simulink model "RealLifeTrainModel"  (R2024a)
settings: Solver=ode1  StartTime=0.0  StopTime=Inf  FixedStep=0.001  RelTol=1e-3
PostLoadFcn:
  | , if any(exist('dsrtsu_mdlpostloadfcn', 'file') ~= 0), dsrtsu_mdlpostloadfcn('Execute', bdroot); end,
InitFcn:
  | , if any(exist('rtifpga_mdlclblib', 'file') ~= 0), rtifpga_mdlclblib('Init', bdroot); end,
undefined symbols (not defined in the file): DiscIntNeverNeededParam
libraries: deeplib x29, svdutilitieslib x28, simulink x8, eeGeneralControl x8, rti1202lib_adc_class1 x6, rti1202serlib x5, spsEdgeDetectorLib x5, rtiemclib x2, rti1202lib_dac_class1 x1
(part 5 of 8)

== system RealLifeTrainModel/ContractionMetricFilterSystem3/Calc_A_B/Calc_A_Grad/IndidualGrad6 ==
  State : Inport
  Position : Inport  Port=2
  StartValue : Inport  Port=3
  Data Type Conversion2 : DataTypeConversion  OutDataTypeStr=single  SaturateOnIntegerOverflow=off  RndMeth=Floor
  Data Type Conversion4 : DataTypeConversion  OutDataTypeStr=single  SaturateOnIntegerOverflow=off  RndMeth=Floor
  DynamicsConvert : MATLAB Function  TreatAsAtomicUnit=on
  MATLAB Function2 : MATLAB Function  TreatAsAtomicUnit=on
  MATLAB Function5 : MATLAB Function  TreatAsAtomicUnit=on
  Reshape : Reshape  OutputDimensionality=Customize  OutputDimensions=[8,1]
  Reshape1 : Reshape  OutputDimensionality=Customize  OutputDimensions=[8,1]
  Reshape2 : Reshape  OutputDimensionality=Customize  OutputDimensions=[8,1]
  SubsystemModel : Subsystem
  Sum4 : Sum  Inputs=|++
  Grad : Outport
  wires:
  [GradConst] -> MATLAB Function5/3(const)
  Sum4/1 -> Data Type Conversion2/1
  [GradConst] -> MATLAB Function2/1(u)
  State/1 -> Sum4/1
  MATLAB Function2/1(y) -> Sum4/2
  Position/1 -> MATLAB Function2/2(pos)
  MATLAB Function5/1(y) -> Reshape2/1
  StartValue/1 -> Reshape1/1
  Data Type Conversion2/1 -> SubsystemModel/1(u), DynamicsConvert/1(x)
  SubsystemModel/1(y) -> Data Type Conversion4/1
  [DiscreteContinousMode] -> DynamicsConvert/3(useDerivative)
  DynamicsConvert/1(dstate) -> Reshape/1
  Data Type Conversion4/1 -> DynamicsConvert/2(y_model)
  Reshape/1 -> MATLAB Function5/1(u1)
  Reshape1/1 -> MATLAB Function5/2(u2)
  Reshape2/1 -> Grad/1

== system RealLifeTrainModel/ContractionMetricFilterSystem3/Calc_A_B/Calc_A_Grad/IndidualGrad7 ==
  State : Inport
  Position : Inport  Port=2
  StartValue : Inport  Port=3
  Data Type Conversion2 : DataTypeConversion  OutDataTypeStr=single  SaturateOnIntegerOverflow=off  RndMeth=Floor
  Data Type Conversion4 : DataTypeConversion  OutDataTypeStr=single  SaturateOnIntegerOverflow=off  RndMeth=Floor
  DynamicsConvert : MATLAB Function  TreatAsAtomicUnit=on
  MATLAB Function2 : MATLAB Function  TreatAsAtomicUnit=on
  MATLAB Function5 : MATLAB Function  TreatAsAtomicUnit=on
  Reshape : Reshape  OutputDimensionality=Customize  OutputDimensions=[8,1]
  Reshape1 : Reshape  OutputDimensionality=Customize  OutputDimensions=[8,1]
  Reshape2 : Reshape  OutputDimensionality=Customize  OutputDimensions=[8,1]
  SubsystemModel : Subsystem
  Sum4 : Sum  Inputs=|++
  Grad : Outport
  wires:
  [GradConst] -> MATLAB Function5/3(const)
  Sum4/1 -> Data Type Conversion2/1
  [GradConst] -> MATLAB Function2/1(u)
  State/1 -> Sum4/1
  MATLAB Function2/1(y) -> Sum4/2
  Position/1 -> MATLAB Function2/2(pos)
  MATLAB Function5/1(y) -> Reshape2/1
  StartValue/1 -> Reshape1/1
  Data Type Conversion2/1 -> SubsystemModel/1(u), DynamicsConvert/1(x)
  SubsystemModel/1(y) -> Data Type Conversion4/1
  [DiscreteContinousMode] -> DynamicsConvert/3(useDerivative)
  Data Type Conversion4/1 -> DynamicsConvert/2(y_model)
  DynamicsConvert/1(dstate) -> Reshape/1
  Reshape/1 -> MATLAB Function5/1(u1)
  Reshape1/1 -> MATLAB Function5/2(u2)
  Reshape2/1 -> Grad/1

== system RealLifeTrainModel/ContractionMetricFilterSystem3/Calc_A_B/Calc_A_Grad/IndidualGrad8 ==
  State : Inport
  Position : Inport  Port=2
  StartValue : Inport  Port=3
  Data Type Conversion2 : DataTypeConversion  OutDataTypeStr=single  SaturateOnIntegerOverflow=off  RndMeth=Floor
  Data Type Conversion4 : DataTypeConversion  OutDataTypeStr=single  SaturateOnIntegerOverflow=off  RndMeth=Floor
  DynamicsConvert1 : MATLAB Function  TreatAsAtomicUnit=on
  MATLAB Function2 : MATLAB Function  TreatAsAtomicUnit=on
  MATLAB Function5 : MATLAB Function  TreatAsAtomicUnit=on
  Reshape : Reshape  OutputDimensionality=Customize  OutputDimensions=[8,1]
  Reshape1 : Reshape  OutputDimensionality=Customize  OutputDimensions=[8,1]
  Reshape2 : Reshape  OutputDimensionality=Customize  OutputDimensions=[8,1]
  SubsystemModel : Subsystem
  Sum4 : Sum  Inputs=|++
  Grad : Outport
  wires:
  [GradConst] -> MATLAB Function5/3(const)
  Sum4/1 -> Data Type Conversion2/1
  [GradConst] -> MATLAB Function2/1(u)
  State/1 -> Sum4/1
  MATLAB Function2/1(y) -> Sum4/2
  Position/1 -> MATLAB Function2/2(pos)
  StartValue/1 -> Reshape2/1
  Data Type Conversion2/1 -> SubsystemModel/1(u), DynamicsConvert1/1(x)
  SubsystemModel/1(y) -> Data Type Conversion4/1
  [DiscreteContinousMode] -> DynamicsConvert1/3(useDerivative)
  Data Type Conversion4/1 -> DynamicsConvert1/2(y_model)
  DynamicsConvert1/1(dstate) -> Reshape1/1
  MATLAB Function5/1(y) -> Reshape/1
  Reshape/1 -> Grad/1
  Reshape1/1 -> MATLAB Function5/1(u1)
  Reshape2/1 -> MATLAB Function5/2(u2)

== system RealLifeTrainModel/ContractionMetricFilterSystem3/Calc_A_B/Calc_A_Grad/SubsystemModel ==
  u : Inport
  Denormalize : MATLAB Function  TreatAsAtomicUnit=on
  Normalize : MATLAB Function  TreatAsAtomicUnit=on
  PredictModel : deeplib/Predict  Network=Network from MAT-file  NetworkFunction=squeezenet  NetworkFilePath=C:\Users\ic2d\Documents\GitHub\dSpace_Controllers_legged\model_1.mat  MiniBatchSize=128  InputDataFormats={'input', 'BC';}  Predictions=on  Activations={}  ForceInterpretedSim=off  EnableDLNetwork=on  LastKnownNetworkFilePath='C:\Users\ic2d\Documents\GitHub\dSpace_Controllers_legged\model_1.mat'  LastKnownNetworkTimeStamp=739864.429490740760229527950286865234375
  PredictModel1 : deeplib/Predict  Network=Network from MAT-file  NetworkFunction=squeezenet  NetworkFilePath=C:\Users\ic2d\Documents\GitHub\dSpace_Controllers_legged\model_2.mat  MiniBatchSize=128  InputDataFormats={'input', 'BC';}  Predictions=on  Activations={}  ForceInterpretedSim=off  EnableDLNetwork=on  LastKnownNetworkFilePath='C:\Users\ic2d\Documents\GitHub\dSpace_Controllers_legged\model_2.mat'  LastKnownNetworkTimeStamp=739864.429490740760229527950286865234375
  Product : Product
  Scope : Scope
  Square : Math  Operator=square
  Subsystem : Subsystem
  Subsystem1 : Subsystem
  Sum : Sum  Inputs=|++
  Transpose : Math  Operator=transpose
  y : Outport
  wires:
  PredictModel1/1 -> Square/1
  Square/1 -> Product/1
  Denormalize/1(y) -> y/1
  PredictModel/1 -> Sum/1
  Product/1 -> Sum/2
  Sum/1 -> Denormalize/1(u)
  u/1 -> Normalize/1(u)
  Normalize/1(y) -> Subsystem1/1(In1), Scope/1, Subsystem/1(In1)
  Subsystem1/1(Out1) -> Product/2
  Transpose/1 -> PredictModel1/1, PredictModel/1
  Subsystem/1(Out1) -> Transpose/1

== system RealLifeTrainModel/RTI Data/RTI Data Store/RTI Data Store/RTI Data Store ==
  RTI Data Store : Subsystem  mask(RTI_DATA_STORE){}
      mask help:
      | RTI Data Store Block. This block is used by RTI to store internal model dependent data. Deleting this block will result in data loss.
      |
      | NEVER DELETE, COPY, OR MODIFY THIS BLOCK!
      mask Help:
      | RTI Data Store Block. This block is used by RTI to store internal model dependent data. Deleting this block will result in data loss.
      | 
      | NEVER DELETE, COPY, OR MODIFY THIS BLOCK!
      mask Display: text(0.5, 0.5, ' ', 'HorizontalAlignment', 'center');

== system RealLifeTrainModel/ContractionMetricFilterSystem3/Calc_A_B/Calc_A_Grad/IndidualGrad1/SubsystemModel ==
  u : Inport
  Denormalize : MATLAB Function  TreatAsAtomicUnit=on
  Normalize : MATLAB Function  TreatAsAtomicUnit=on
  PredictModel : deeplib/Predict  Network=Network from MAT-file  NetworkFunction=squeezenet  NetworkFilePath=C:\Users\ic2d\Documents\GitHub\dSpace_Controllers_legged\model_1.mat  MiniBatchSize=128  InputDataFormats={'input', 'BC';}  Predictions=on  Activations={}  ForceInterpretedSim=off  EnableDLNetwork=on  LastKnownNetworkFilePath='C:\Users\ic2d\Documents\GitHub\dSpace_Controllers_legged\model_1.mat'  LastKnownNetworkTimeStamp=739864.429490740760229527950286865234375
  PredictModel1 : deeplib/Predict  Network=Network from MAT-file  NetworkFunction=squeezenet  NetworkFilePath=C:\Users\ic2d\Documents\GitHub\dSpace_Controllers_legged\model_2.mat  MiniBatchSize=128  InputDataFormats={'input', 'BC';}  Predictions=on  Activations={}  ForceInterpretedSim=off  EnableDLNetwork=on  LastKnownNetworkFilePath='C:\Users\ic2d\Documents\GitHub\dSpace_Controllers_legged\model_2.mat'  LastKnownNetworkTimeStamp=739864.429490740760229527950286865234375
  Product : Product
  Square : Math  Operator=square
  Subsystem : Subsystem
  Subsystem1 : Subsystem
  Sum : Sum  Inputs=|++
  Transpose : Math  Operator=transpose
  y : Outport
  wires:
  PredictModel1/1 -> Square/1
  Square/1 -> Product/1
  Denormalize/1(y) -> y/1
  PredictModel/1 -> Sum/1
  Product/1 -> Sum/2
  Sum/1 -> Denormalize/1(u)
  u/1 -> Normalize/1(u)
  Normalize/1(y) -> Subsystem1/1(In1), Subsystem/1(In1)
  Subsystem/1(Out1) -> Transpose/1
  Subsystem1/1(Out1) -> Product/2
  Transpose/1 -> PredictModel1/1, PredictModel/1

== system RealLifeTrainModel/ContractionMetricFilterSystem3/Calc_A_B/Calc_A_Grad/IndidualGrad10/SubsystemModel ==
  u : Inport
  Denormalize : MATLAB Function  TreatAsAtomicUnit=on
  Normalize : MATLAB Function  TreatAsAtomicUnit=on
  PredictModel : deeplib/Predict  Network=Network from MAT-file  NetworkFunction=squeezenet  NetworkFilePath=C:\Users\ic2d\Documents\GitHub\dSpace_Controllers_legged\model_1.mat  MiniBatchSize=128  InputDataFormats={'input', 'BC';}  Predictions=on  Activations={}  ForceInterpretedSim=off  EnableDLNetwork=on  LastKnownNetworkFilePath='C:\Users\ic2d\Documents\GitHub\dSpace_Controllers_legged\model_1.mat'  LastKnownNetworkTimeStamp=739864.429490740760229527950286865234375
  PredictModel1 : deeplib/Predict  Network=Network from MAT-file  NetworkFunction=squeezenet  NetworkFilePath=C:\Users\ic2d\Documents\GitHub\dSpace_Controllers_legged\model_2.mat  MiniBatchSize=128  InputDataFormats={'input', 'BC';}  Predictions=on  Activations={}  ForceInterpretedSim=off  EnableDLNetwork=on  LastKnownNetworkFilePath='C:\Users\ic2d\Documents\GitHub\dSpace_Controllers_legged\model_2.mat'  LastKnownNetworkTimeStamp=739864.429490740760229527950286865234375
  Product : Product
  Square : Math  Operator=square
  Subsystem : Subsystem
  Subsystem1 : Subsystem
  Sum : Sum  Inputs=|++
  Transpose : Math  Operator=transpose
  y : Outport
  wires:
  PredictModel1/1 -> Square/1
  Square/1 -> Product/1
  Denormalize/1(y) -> y/1
  PredictModel/1 -> Sum/1
  Product/1 -> Sum/2
  Sum/1 -> Denormalize/1(u)
  u/1 -> Normalize/1(u)
  Normalize/1(y) -> Subsystem1/1(In1), Subsystem/1(In1)
  Subsystem/1(Out1) -> Transpose/1
  Subsystem1/1(Out1) -> Product/2
  Transpose/1 -> PredictModel1/1, PredictModel/1

== system RealLifeTrainModel/ContractionMetricFilterSystem3/Calc_A_B/Calc_A_Grad/IndidualGrad2/SubsystemModel ==
  u : Inport
  Denormalize : MATLAB Function  TreatAsAtomicUnit=on
  Normalize : MATLAB Function  TreatAsAtomicUnit=on
  PredictModel : deeplib/Predict  Network=Network from MAT-file  NetworkFunction=squeezenet  NetworkFilePath=C:\Users\ic2d\Documents\GitHub\dSpace_Controllers_legged\model_1.mat  MiniBatchSize=128  InputDataFormats={'input', 'BC';}  Predictions=on  Activations={}  ForceInterpretedSim=off  EnableDLNetwork=on  LastKnownNetworkFilePath='C:\Users\ic2d\Documents\GitHub\dSpace_Controllers_legged\model_1.mat'  LastKnownNetworkTimeStamp=739864.429490740760229527950286865234375
  PredictModel1 : deeplib/Predict  Network=Network from MAT-file  NetworkFunction=squeezenet  NetworkFilePath=C:\Users\ic2d\Documents\GitHub\dSpace_Controllers_legged\model_2.mat  MiniBatchSize=128  InputDataFormats={'input', 'BC';}  Predictions=on  Activations={}  ForceInterpretedSim=off  EnableDLNetwork=on  LastKnownNetworkFilePath='C:\Users\ic2d\Documents\GitHub\dSpace_Controllers_legged\model_2.mat'  LastKnownNetworkTimeStamp=739864.429490740760229527950286865234375
  Product : Product
  Square : Math  Operator=square
  Subsystem : Subsystem
  Subsystem1 : Subsystem
  Sum : Sum  Inputs=|++
  Transpose : Math  Operator=transpose
  y : Outport
  wires:
  PredictModel1/1 -> Square/1
  Square/1 -> Product/1
  Denormalize/1(y) -> y/1
  PredictModel/1 -> Sum/1
  Product/1 -> Sum/2
  Sum/1 -> Denormalize/1(u)
  u/1 -> Normalize/1(u)
  Normalize/1(y) -> Subsystem1/1(In1), Subsystem/1(In1)
  Subsystem/1(Out1) -> Transpose/1
  Subsystem1/1(Out1) -> Product/2
  Transpose/1 -> PredictModel1/1, PredictModel/1

== system RealLifeTrainModel/ContractionMetricFilterSystem3/Calc_A_B/Calc_A_Grad/IndidualGrad3/SubsystemModel ==
  u : Inport
  Denormalize : MATLAB Function  TreatAsAtomicUnit=on
  Normalize : MATLAB Function  TreatAsAtomicUnit=on
  PredictModel : deeplib/Predict  Network=Network from MAT-file  NetworkFunction=squeezenet  NetworkFilePath=C:\Users\ic2d\Documents\GitHub\dSpace_Controllers_legged\model_1.mat  MiniBatchSize=128  InputDataFormats={'input', 'BC';}  Predictions=on  Activations={}  ForceInterpretedSim=off  EnableDLNetwork=on  LastKnownNetworkFilePath='C:\Users\ic2d\Documents\GitHub\dSpace_Controllers_legged\model_1.mat'  LastKnownNetworkTimeStamp=739864.429490740760229527950286865234375
  PredictModel1 : deeplib/Predict  Network=Network from MAT-file  NetworkFunction=squeezenet  NetworkFilePath=C:\Users\ic2d\Documents\GitHub\dSpace_Controllers_legged\model_2.mat  MiniBatchSize=128  InputDataFormats={'input', 'BC';}  Predictions=on  Activations={}  ForceInterpretedSim=off  EnableDLNetwork=on  LastKnownNetworkFilePath='C:\Users\ic2d\Documents\GitHub\dSpace_Controllers_legged\model_2.mat'  LastKnownNetworkTimeStamp=739864.429490740760229527950286865234375
  Product : Product
  Square : Math  Operator=square
  Subsystem : Subsystem
  Subsystem1 : Subsystem
  Sum : Sum  Inputs=|++
  Transpose : Math  Operator=transpose
  y : Outport
  wires:
  PredictModel1/1 -> Square/1
  Square/1 -> Product/1
  Denormalize/1(y) -> y/1
  PredictModel/1 -> Sum/1
  Product/1 -> Sum/2
  Sum/1 -> Denormalize/1(u)
  u/1 -> Normalize/1(u)
  Normalize/1(y) -> Subsystem1/1(In1), Subsystem/1(In1)
  Subsystem/1(Out1) -> Transpose/1
  Subsystem1/1(Out1) -> Product/2
  Transpose/1 -> PredictModel1/1, PredictModel/1

== system RealLifeTrainModel/ContractionMetricFilterSystem3/Calc_A_B/Calc_A_Grad/IndidualGrad4/SubsystemModel ==
  u : Inport
  Denormalize : MATLAB Function  TreatAsAtomicUnit=on
  Normalize : MATLAB Function  TreatAsAtomicUnit=on
  PredictModel : deeplib/Predict  Network=Network from MAT-file  NetworkFunction=squeezenet  NetworkFilePath=C:\Users\ic2d\Documents\GitHub\dSpace_Controllers_legged\model_1.mat  MiniBatchSize=128  InputDataFormats={'input', 'BC';}  Predictions=on  Activations={}  ForceInterpretedSim=off  EnableDLNetwork=on  LastKnownNetworkFilePath='C:\Users\ic2d\Documents\GitHub\dSpace_Controllers_legged\model_1.mat'  LastKnownNetworkTimeStamp=739864.429490740760229527950286865234375
  PredictModel1 : deeplib/Predict  Network=Network from MAT-file  NetworkFunction=squeezenet  NetworkFilePath=C:\Users\ic2d\Documents\GitHub\dSpace_Controllers_legged\model_2.mat  MiniBatchSize=128  InputDataFormats={'input', 'BC';}  Predictions=on  Activations={}  ForceInterpretedSim=off  EnableDLNetwork=on  LastKnownNetworkFilePath='C:\Users\ic2d\Documents\GitHub\dSpace_Controllers_legged\model_2.mat'  LastKnownNetworkTimeStamp=739864.429490740760229527950286865234375
  Product : Product
  Square : Math  Operator=square
  Subsystem : Subsystem
  Subsystem1 : Subsystem
  Sum : Sum  Inputs=|++
  Transpose : Math  Operator=transpose
  y : Outport
  wires:
  PredictModel1/1 -> Square/1
  Square/1 -> Product/1
  Denormalize/1(y) -> y/1
  PredictModel/1 -> Sum/1
  Product/1 -> Sum/2
  Sum/1 -> Denormalize/1(u)
  u/1 -> Normalize/1(u)
  Normalize/1(y) -> Subsystem1/1(In1), Subsystem/1(In1)
  Subsystem/1(Out1) -> Transpose/1
  Subsystem1/1(Out1) -> Product/2
  Transpose/1 -> PredictModel1/1, PredictModel/1

== system RealLifeTrainModel/ContractionMetricFilterSystem3/Calc_A_B/Calc_A_Grad/IndidualGrad5/SubsystemModel ==
  u : Inport
  Denormalize : MATLAB Function  TreatAsAtomicUnit=on
  Normalize : MATLAB Function  TreatAsAtomicUnit=on
  PredictModel : deeplib/Predict  Network=Network from MAT-file  NetworkFunction=squeezenet  NetworkFilePath=C:\Users\ic2d\Documents\GitHub\dSpace_Controllers_legged\model_1.mat  MiniBatchSize=128  InputDataFormats={'input', 'BC';}  Predictions=on  Activations={}  ForceInterpretedSim=off  EnableDLNetwork=on  LastKnownNetworkFilePath='C:\Users\ic2d\Documents\GitHub\dSpace_Controllers_legged\model_1.mat'  LastKnownNetworkTimeStamp=739864.429490740760229527950286865234375
  PredictModel1 : deeplib/Predict  Network=Network from MAT-file  NetworkFunction=squeezenet  NetworkFilePath=C:\Users\ic2d\Documents\GitHub\dSpace_Controllers_legged\model_2.mat  MiniBatchSize=128  InputDataFormats={'input', 'BC';}  Predictions=on  Activations={}  ForceInterpretedSim=off  EnableDLNetwork=on  LastKnownNetworkFilePath='C:\Users\ic2d\Documents\GitHub\dSpace_Controllers_legged\model_2.mat'  LastKnownNetworkTimeStamp=739864.429490740760229527950286865234375
  Product : Product
  Square : Math  Operator=square
  Subsystem : Subsystem
  Subsystem1 : Subsystem
  Sum : Sum  Inputs=|++
  Transpose : Math  Operator=transpose
  y : Outport
  wires:
  PredictModel1/1 -> Square/1
  Square/1 -> Product/1
  Denormalize/1(y) -> y/1
  PredictModel/1 -> Sum/1
  Product/1 -> Sum/2
  Sum/1 -> Denormalize/1(u)
  u/1 -> Normalize/1(u)
  Normalize/1(y) -> Subsystem1/1(In1), Subsystem/1(In1)
  Subsystem/1(Out1) -> Transpose/1
  Subsystem1/1(Out1) -> Product/2
  Transpose/1 -> PredictModel1/1, PredictModel/1

== system RealLifeTrainModel/ContractionMetricFilterSystem3/Calc_A_B/Calc_A_Grad/IndidualGrad6/SubsystemModel ==
  u : Inport
  Denormalize : MATLAB Function  TreatAsAtomicUnit=on
  Normalize : MATLAB Function  TreatAsAtomicUnit=on
  PredictModel : deeplib/Predict  Network=Network from MAT-file  NetworkFunction=squeezenet  NetworkFilePath=C:\Users\ic2d\Documents\GitHub\dSpace_Controllers_legged\model_1.mat  MiniBatchSize=128  InputDataFormats={'input', 'BC';}  Predictions=on  Activations={}  ForceInterpretedSim=off  EnableDLNetwork=on  LastKnownNetworkFilePath='C:\Users\ic2d\Documents\GitHub\dSpace_Controllers_legged\model_1.mat'  LastKnownNetworkTimeStamp=739864.429490740760229527950286865234375
  PredictModel1 : deeplib/Predict  Network=Network from MAT-file  NetworkFunction=squeezenet  NetworkFilePath=C:\Users\ic2d\Documents\GitHub\dSpace_Controllers_legged\model_2.mat  MiniBatchSize=128  InputDataFormats={'input', 'BC';}  Predictions=on  Activations={}  ForceInterpretedSim=off  EnableDLNetwork=on  LastKnownNetworkFilePath='C:\Users\ic2d\Documents\GitHub\dSpace_Controllers_legged\model_2.mat'  LastKnownNetworkTimeStamp=739864.429490740760229527950286865234375
  Product : Product
  Square : Math  Operator=square
  Subsystem : Subsystem
  Subsystem1 : Subsystem
  Sum : Sum  Inputs=|++
  Transpose : Math  Operator=transpose
  y : Outport
  wires:
  PredictModel1/1 -> Square/1
  Square/1 -> Product/1
  Denormalize/1(y) -> y/1
  PredictModel/1 -> Sum/1
  Product/1 -> Sum/2
  Sum/1 -> Denormalize/1(u)
  u/1 -> Normalize/1(u)
  Normalize/1(y) -> Subsystem1/1(In1), Subsystem/1(In1)
  Subsystem/1(Out1) -> Transpose/1
  Subsystem1/1(Out1) -> Product/2
  Transpose/1 -> PredictModel1/1, PredictModel/1

== system RealLifeTrainModel/ContractionMetricFilterSystem3/Calc_A_B/Calc_A_Grad/IndidualGrad7/SubsystemModel ==
  u : Inport
  Denormalize : MATLAB Function  TreatAsAtomicUnit=on
  Normalize : MATLAB Function  TreatAsAtomicUnit=on
  PredictModel : deeplib/Predict  Network=Network from MAT-file  NetworkFunction=squeezenet  NetworkFilePath=C:\Users\ic2d\Documents\GitHub\dSpace_Controllers_legged\model_1.mat  MiniBatchSize=128  InputDataFormats={'input', 'BC';}  Predictions=on  Activations={}  ForceInterpretedSim=off  EnableDLNetwork=on  LastKnownNetworkFilePath='C:\Users\ic2d\Documents\GitHub\dSpace_Controllers_legged\model_1.mat'  LastKnownNetworkTimeStamp=739864.429490740760229527950286865234375
  PredictModel1 : deeplib/Predict  Network=Network from MAT-file  NetworkFunction=squeezenet  NetworkFilePath=C:\Users\ic2d\Documents\GitHub\dSpace_Controllers_legged\model_2.mat  MiniBatchSize=128  InputDataFormats={'input', 'BC';}  Predictions=on  Activations={}  ForceInterpretedSim=off  EnableDLNetwork=on  LastKnownNetworkFilePath='C:\Users\ic2d\Documents\GitHub\dSpace_Controllers_legged\model_2.mat'  LastKnownNetworkTimeStamp=739864.429490740760229527950286865234375
  Product : Product
  Square : Math  Operator=square
  Subsystem : Subsystem
  Subsystem1 : Subsystem
  Sum : Sum  Inputs=|++
  Transpose : Math  Operator=transpose
  y : Outport
  wires:
  PredictModel1/1 -> Square/1
  Square/1 -> Product/1
  Denormalize/1(y) -> y/1
  PredictModel/1 -> Sum/1
  Product/1 -> Sum/2
  Sum/1 -> Denormalize/1(u)
  u/1 -> Normalize/1(u)
  Normalize/1(y) -> Subsystem1/1(In1), Subsystem/1(In1)
  Subsystem/1(Out1) -> Transpose/1
  Subsystem1/1(Out1) -> Product/2
  Transpose/1 -> PredictModel1/1, PredictModel/1

== system RealLifeTrainModel/ContractionMetricFilterSystem3/Calc_A_B/Calc_A_Grad/IndidualGrad8/SubsystemModel ==
  u : Inport
  Denormalize : MATLAB Function  TreatAsAtomicUnit=on
  Normalize : MATLAB Function  TreatAsAtomicUnit=on
  PredictModel : deeplib/Predict  Network=Network from MAT-file  NetworkFunction=squeezenet  NetworkFilePath=C:\Users\ic2d\Documents\GitHub\dSpace_Controllers_legged\model_1.mat  MiniBatchSize=128  InputDataFormats={'input', 'BC';}  Predictions=on  Activations={}  ForceInterpretedSim=off  EnableDLNetwork=on  LastKnownNetworkFilePath='C:\Users\ic2d\Documents\GitHub\dSpace_Controllers_legged\model_1.mat'  LastKnownNetworkTimeStamp=739864.429490740760229527950286865234375
  PredictModel1 : deeplib/Predict  Network=Network from MAT-file  NetworkFunction=squeezenet  NetworkFilePath=C:\Users\ic2d\Documents\GitHub\dSpace_Controllers_legged\model_2.mat  MiniBatchSize=128  InputDataFormats={'input', 'BC';}  Predictions=on  Activations={}  ForceInterpretedSim=off  EnableDLNetwork=on  LastKnownNetworkFilePath='C:\Users\ic2d\Documents\GitHub\dSpace_Controllers_legged\model_2.mat'  LastKnownNetworkTimeStamp=739864.429490740760229527950286865234375
  Product : Product
  Square : Math  Operator=square
  Subsystem : Subsystem
  Subsystem1 : Subsystem
  Sum : Sum  Inputs=|++
  Transpose : Math  Operator=transpose
  y : Outport
  wires:
  PredictModel1/1 -> Square/1
  Square/1 -> Product/1
  Denormalize/1(y) -> y/1
  PredictModel/1 -> Sum/1
  Product/1 -> Sum/2
  Sum/1 -> Denormalize/1(u)
  u/1 -> Normalize/1(u)
  Normalize/1(y) -> Subsystem1/1(In1), Subsystem/1(In1)
  Subsystem1/1(Out1) -> Product/2
  Subsystem/1(Out1) -> Transpose/1
  Transpose/1 -> PredictModel1/1, PredictModel/1

== system RealLifeTrainModel/ContractionMetricFilterSystem3/Calc_A_B/Calc_A_Grad/SubsystemModel/Subsystem ==
  In1 : Inport
  Demux : Demux  Outputs=9
  Mux : Mux  Inputs=8
  Out1 : Outport
  wires:
  In1/1 -> Demux/1
  Demux/1 -> Mux/1
  Demux/2 -> Mux/2
  Demux/3 -> Mux/3
  Demux/4 -> Mux/4
  Demux/5 -> Mux/5
  Demux/6 -> Mux/6
  Demux/7 -> Mux/7
  Demux/8 -> Mux/8
  Mux/1 -> Out1/1

== system RealLifeTrainModel/ContractionMetricFilterSystem3/Calc_A_B/Calc_A_Grad/SubsystemModel/Subsystem1 ==
  In1 : Inport
  Demux : Demux  Outputs=9
  Out1 : Outport
  wires:
  In1/1 -> Demux/1
  Demux/9 -> Out1/1

== system RealLifeTrainModel/RTI Data/RTI Data Store/RTI Data Store/RTI Data Store/RTI Data Store ==

== system RealLifeTrainModel/ContractionMetricFilterSystem3/Calc_A_B/Calc_A_Grad/IndidualGrad1/SubsystemModel/Subsystem ==
  In1 : Inport
  Demux : Demux  Outputs=9
  Mux : Mux  Inputs=8
  Out1 : Outport
  wires:
  In1/1 -> Demux/1
  Demux/1 -> Mux/1
  Demux/2 -> Mux/2
  Demux/3 -> Mux/3
  Demux/4 -> Mux/4
  Demux/5 -> Mux/5
  Demux/6 -> Mux/6
  Demux/7 -> Mux/7
  Demux/8 -> Mux/8
  Mux/1 -> Out1/1

== system RealLifeTrainModel/ContractionMetricFilterSystem3/Calc_A_B/Calc_A_Grad/IndidualGrad1/SubsystemModel/Subsystem1 ==
  In1 : Inport
  Demux : Demux  Outputs=9
  Out1 : Outport
  wires:
  In1/1 -> Demux/1
  Demux/9 -> Out1/1

== system RealLifeTrainModel/ContractionMetricFilterSystem3/Calc_A_B/Calc_A_Grad/IndidualGrad10/SubsystemModel/Subsystem ==
  In1 : Inport
  Demux : Demux  Outputs=9
  Mux : Mux  Inputs=8
  Out1 : Outport
  wires:
  In1/1 -> Demux/1
  Demux/1 -> Mux/1
  Demux/2 -> Mux/2
  Demux/3 -> Mux/3
  Demux/4 -> Mux/4
  Demux/5 -> Mux/5
  Demux/6 -> Mux/6
  Demux/7 -> Mux/7
  Demux/8 -> Mux/8
  Mux/1 -> Out1/1

== system RealLifeTrainModel/ContractionMetricFilterSystem3/Calc_A_B/Calc_A_Grad/IndidualGrad10/SubsystemModel/Subsystem1 ==
  In1 : Inport
  Demux : Demux  Outputs=9
  Out1 : Outport
  wires:
  In1/1 -> Demux/1
  Demux/9 -> Out1/1

== system RealLifeTrainModel/ContractionMetricFilterSystem3/Calc_A_B/Calc_A_Grad/IndidualGrad2/SubsystemModel/Subsystem ==
  In1 : Inport
  Demux : Demux  Outputs=9
  Mux : Mux  Inputs=8
  Out1 : Outport
  wires:
  In1/1 -> Demux/1
  Demux/1 -> Mux/1
  Demux/2 -> Mux/2
  Demux/3 -> Mux/3
  Demux/4 -> Mux/4
  Demux/5 -> Mux/5
  Demux/6 -> Mux/6
  Demux/7 -> Mux/7
  Demux/8 -> Mux/8
  Mux/1 -> Out1/1

== system RealLifeTrainModel/ContractionMetricFilterSystem3/Calc_A_B/Calc_A_Grad/IndidualGrad2/SubsystemModel/Subsystem1 ==
  In1 : Inport
  Demux : Demux  Outputs=9
  Out1 : Outport
  wires:
  In1/1 -> Demux/1
  Demux/9 -> Out1/1

== system RealLifeTrainModel/ContractionMetricFilterSystem3/Calc_A_B/Calc_A_Grad/IndidualGrad3/SubsystemModel/Subsystem ==
  In1 : Inport
  Demux : Demux  Outputs=9
  Mux : Mux  Inputs=8
  Out1 : Outport
  wires:
  In1/1 -> Demux/1
  Demux/1 -> Mux/1
  Demux/2 -> Mux/2
  Demux/3 -> Mux/3
  Demux/4 -> Mux/4
  Demux/5 -> Mux/5
  Demux/6 -> Mux/6
  Demux/7 -> Mux/7
  Demux/8 -> Mux/8
  Mux/1 -> Out1/1

== system RealLifeTrainModel/ContractionMetricFilterSystem3/Calc_A_B/Calc_A_Grad/IndidualGrad3/SubsystemModel/Subsystem1 ==
  In1 : Inport
  Demux : Demux  Outputs=9
  Out1 : Outport
  wires:
  In1/1 -> Demux/1
  Demux/9 -> Out1/1

== system RealLifeTrainModel/ContractionMetricFilterSystem3/Calc_A_B/Calc_A_Grad/IndidualGrad4/SubsystemModel/Subsystem ==
  In1 : Inport
  Demux : Demux  Outputs=9
  Mux : Mux  Inputs=8
  Out1 : Outport
  wires:
  In1/1 -> Demux/1
  Demux/1 -> Mux/1
  Demux/2 -> Mux/2
  Demux/3 -> Mux/3
  Demux/4 -> Mux/4
  Demux/5 -> Mux/5
  Demux/6 -> Mux/6
  Demux/7 -> Mux/7
  Demux/8 -> Mux/8
  Mux/1 -> Out1/1

== system RealLifeTrainModel/ContractionMetricFilterSystem3/Calc_A_B/Calc_A_Grad/IndidualGrad4/SubsystemModel/Subsystem1 ==
  In1 : Inport
  Demux : Demux  Outputs=9
  Out1 : Outport
  wires:
  In1/1 -> Demux/1
  Demux/9 -> Out1/1

== system RealLifeTrainModel/ContractionMetricFilterSystem3/Calc_A_B/Calc_A_Grad/IndidualGrad5/SubsystemModel/Subsystem ==
  In1 : Inport
  Demux : Demux  Outputs=9
  Mux : Mux  Inputs=8
  Out1 : Outport
  wires:
  In1/1 -> Demux/1
  Demux/1 -> Mux/1
  Demux/2 -> Mux/2
  Demux/3 -> Mux/3
  Demux/4 -> Mux/4
  Demux/5 -> Mux/5
  Demux/6 -> Mux/6
  Demux/7 -> Mux/7
  Demux/8 -> Mux/8
  Mux/1 -> Out1/1

== system RealLifeTrainModel/ContractionMetricFilterSystem3/Calc_A_B/Calc_A_Grad/IndidualGrad5/SubsystemModel/Subsystem1 ==
  In1 : Inport
  Demux : Demux  Outputs=9
  Out1 : Outport
  wires:
  In1/1 -> Demux/1
  Demux/9 -> Out1/1

== system RealLifeTrainModel/ContractionMetricFilterSystem3/Calc_A_B/Calc_A_Grad/IndidualGrad6/SubsystemModel/Subsystem ==
  In1 : Inport
  Demux : Demux  Outputs=9
  Mux : Mux  Inputs=8
  Out1 : Outport
  wires:
  In1/1 -> Demux/1
  Demux/1 -> Mux/1
  Demux/2 -> Mux/2
  Demux/3 -> Mux/3
  Demux/4 -> Mux/4
  Demux/5 -> Mux/5
  Demux/6 -> Mux/6
  Demux/7 -> Mux/7
  Demux/8 -> Mux/8
  Mux/1 -> Out1/1

== system RealLifeTrainModel/ContractionMetricFilterSystem3/Calc_A_B/Calc_A_Grad/IndidualGrad6/SubsystemModel/Subsystem1 ==
  In1 : Inport
  Demux : Demux  Outputs=9
  Out1 : Outport
  wires:
  In1/1 -> Demux/1
  Demux/9 -> Out1/1

== system RealLifeTrainModel/ContractionMetricFilterSystem3/Calc_A_B/Calc_A_Grad/IndidualGrad7/SubsystemModel/Subsystem ==
  In1 : Inport
  Demux : Demux  Outputs=9
  Mux : Mux  Inputs=8
  Out1 : Outport
  wires:
  In1/1 -> Demux/1
  Demux/1 -> Mux/1
  Demux/2 -> Mux/2
  Demux/3 -> Mux/3
  Demux/4 -> Mux/4
  Demux/5 -> Mux/5
  Demux/6 -> Mux/6
  Demux/7 -> Mux/7
  Demux/8 -> Mux/8
  Mux/1 -> Out1/1

== system RealLifeTrainModel/ContractionMetricFilterSystem3/Calc_A_B/Calc_A_Grad/IndidualGrad7/SubsystemModel/Subsystem1 ==
  In1 : Inport
  Demux : Demux  Outputs=9
  Out1 : Outport
  wires:
  In1/1 -> Demux/1
  Demux/9 -> Out1/1

== system RealLifeTrainModel/ContractionMetricFilterSystem3/Calc_A_B/Calc_A_Grad/IndidualGrad8/SubsystemModel/Subsystem ==
  In1 : Inport
  Demux : Demux  Outputs=9
  Mux : Mux  Inputs=8
  Out1 : Outport
  wires:
  In1/1 -> Demux/1
  Demux/1 -> Mux/1
  Demux/2 -> Mux/2
  Demux/3 -> Mux/3
  Demux/4 -> Mux/4
  Demux/5 -> Mux/5
  Demux/6 -> Mux/6
  Demux/7 -> Mux/7
  Demux/8 -> Mux/8
  Mux/1 -> Out1/1

== system RealLifeTrainModel/ContractionMetricFilterSystem3/Calc_A_B/Calc_A_Grad/IndidualGrad8/SubsystemModel/Subsystem1 ==
  In1 : Inport
  Demux : Demux  Outputs=9
  Out1 : Outport
  wires:
  In1/1 -> Demux/1
  Demux/9 -> Out1/1

== matlab function RealLifeTrainModel/ContractionMetricFilterSystem3/CalcK/IndidualGrad1/Policy_SS1/Policy ==
  data: u input; y output
function y = fcn(u)

y = (u)/2 + 0.5;

== matlab function RealLifeTrainModel/ContractionMetricFilterSystem3/CalcK/IndidualGrad1/Policy_SS1/SmoothFnc1 ==
  data: u input; y output; smooth input
function y = fcn(u,smooth)
persistent last_value;

if(isempty(last_value))
    last_value = 0
end

y = smooth*last_value + (1 - smooth)*u
last_value = u

== matlab function RealLifeTrainModel/RefStepFunction ==
  data: Time input; y output; Amp input; StartTime input; EndTime input
function y = fcn(Time,Amp,StartTime,EndTime)

if((Time - StartTime) < 5)
    y = 0;
elseif ((EndTime + StartTime - Time) < 5)
    y = 0;
else
    y = Amp;
end

== matlab function RealLifeTrainModel/ContractionMetricFilterSystem3/CalcK/IndidualGrad10/MATLAB Function2 ==
  data: u input; y output; pos input
function y = fcn(u,pos)

a = [0,0,0,0,0,0,0,0,0]

a(pos) = u

y = a;

== matlab function RealLifeTrainModel/ContractionMetricFilterSystem3/CalcK/IndidualGrad10/MATLAB Function5 ==
  data: u1 input; y output; u2 input; const input
function y = fcn(u1,u2,const)

y = (u1 - u2)/(const);

== matlab function RealLifeTrainModel/ContractionMetricFilterSystem3/CalcK/IndidualGrad10/Policy_SS1/Denormalize_Policy ==
  data: u input; y output
function y = fcn(u)

max_Fload =  569.629505294963
min_Fload = -610.339671010468

max_Fhyd = 729.261146885585
min_Fhyd = -777.489547410502

max_DFload = 123011.265014651
min_DFload = -142353.177843906

max_DFhyd = 219994.429294316
min_DFhyd = -270882.694509076

max_Pa = 12037835.3221229
min_Pa = 1849925.22965178

max_Pb = 14831789.6053956
min_Pb = 2808786.27887814

max_x = 0.082368752
min_x = 0.01990812

max_Dx = 0.682789396628826
min_Dx = -0.578996654196926

out = [1,1,1,1,1,1,1,1,1]

out(1) = (u(1))*(max_Fhyd - min_Fhyd) + min_Fhyd;

out(2) = (u(2))*(max_DFhyd - min_DFhyd) + min_DFhyd;

out(3) = (u(3))*(max_Fload - min_Fload) + min_Fload;

out(4) = (u(4))*(max_DFload - min_DFload) + min_DFload;

out(5) = (u(5))*(max_Pa - min_Pa) + min_Pa;

out(6) = (u(6))*(max_Pb - min_Pb) + min_Pb;

out(7) = (u(7))*(max_x - min_x) + min_x;

out(8) = (u(8))*(max_Dx - min_Dx) + min_Dx;

out(9) = (u(9))*(max_Fload - min_Fload) + min_Fload;


y = out;

== matlab function RealLifeTrainModel/ContractionMetricFilterSystem3/CalcK/IndidualGrad10/Policy_SS1/FLcontroller1 ==
  data: pid input; y output; f input; g input; dFref input; d input; flag_start input
function y = fcn(pid,f,g,dFref,d,flag_start)

if flag_start == 1
    y = (dFref + pid - f)/g - d;
else 
    y = 1;
end

== matlab function RealLifeTrainModel/ContractionMetricFilterSystem3/CalcK/IndidualGrad10/Policy_SS1/FunctionCalculateHydModel1 ==
  data: ixv input; f output; Pn input; Qn input; Un input; Vpl input; Ps input; Pt input; L_cyl input; Aa input; alfa input; c1 input; c2 input; Be input; flag_start input; data input; g output; force output
function [f,g,force] = fcn(ixv,Pn,Qn,Un,Vpl,Ps,Pt,L_cyl,Aa,alfa,c1,c2,Be,flag_start,data)
force = 0
if flag_start == 1
    Pa = data(5)
    Pb = data(6)
    xp = data(7)
    xpd = data(8)
    force = data(3)

    Kv = Qn/(Un*sqrt(Pn/2));
    
    Va = Vpl + Aa*xp;
    Vb = Vpl + (L_cyl - xp)*alfa*Aa;

    if(ixv >= 0)
        g = Be*Aa*Kv*( sign(Ps-Pa)*sqrt(abs(Ps-Pa))/Va + alfa*sign(Pb-Pt)*sqrt(abs(Pb-Pt))/Vb);
    else
        g = Be*Aa*Kv*( sign(Pa-Pt)*sqrt(abs(Pa-Pt))/Va + alfa*sign(Ps-Pb)*sqrt(abs(Ps-Pb))/Vb);
    end
    
    %g1 = Be*Aa*Kv*( sign(Ps-Pa)*sqrt(abs(Ps-Pa))/Va + alfa*sign(Pb-Pt)*sqrt(abs(Pb-Pt))/Vb);
    %g2 = Be*Aa*Kv*( sign(Pa-Pt)*sqrt(abs(Pa-Pt))/Va + alfa*sign(Ps-Pb)*sqrt(abs(Ps-Pb))/Vb);
    %g = (g1 + g2)/2;

    f = -Be*Aa^2*(((alfa)^2)/Vb + 1/Va)*xpd;
    
    g = c2*g;
    f = c1*f;
    
else
    f = 1;
    g = 1;
end

== matlab function RealLifeTrainModel/ContractionMetricFilterSystem3/CalcK/IndidualGrad10/Policy_SS1/Policy ==
  data: u input; y output
function y = fcn(u)

y = (u)/2 + 0.5;

== matlab function RealLifeTrainModel/ContractionMetricFilterSystem3/CalcK/IndidualGrad10/Policy_SS1/SmoothFnc1 ==
  data: u input; y output; smooth input
function y = fcn(u,smooth)
persistent last_value;

if(isempty(last_value))
    last_value = 0
end

y = smooth*last_value + (1 - smooth)*u
last_value = u

== matlab function RealLifeTrainModel/ContractionMetricFilterSystem3/CalcK/IndidualGrad2/MATLAB Function2 ==
  data: u input; y output; pos input
function y = fcn(u,pos)

a = [0,0,0,0,0,0,0,0,0]

a(pos) = u

y = a;

== matlab function RealLifeTrainModel/ContractionMetricFilterSystem3/CalcK/IndidualGrad2/MATLAB Function5 ==
  data: u1 input; y output; u2 input; const input
function y = fcn(u1,u2,const)

y = (u1 - u2)/(const);

== matlab function RealLifeTrainModel/ContractionMetricFilterSystem3/CalcK/IndidualGrad2/Policy_SS1/Denormalize_Policy ==
  data: u input; y output
function y = fcn(u)

max_Fload =  569.629505294963
min_Fload = -610.339671010468

max_Fhyd = 729.261146885585
min_Fhyd = -777.489547410502

max_DFload = 123011.265014651
min_DFload = -142353.177843906

max_DFhyd = 219994.429294316
min_DFhyd = -270882.694509076

max_Pa = 12037835.3221229
min_Pa = 1849925.22965178

max_Pb = 14831789.6053956
min_Pb = 2808786.27887814

max_x = 0.082368752
min_x = 0.01990812

max_Dx = 0.682789396628826
min_Dx = -0.578996654196926

out = [1,1,1,1,1,1,1,1,1]

out(1) = (u(1))*(max_Fhyd - min_Fhyd) + min_Fhyd;

out(2) = (u(2))*(max_DFhyd - min_DFhyd) + min_DFhyd;

out(3) = (u(3))*(max_Fload - min_Fload) + min_Fload;

out(4) = (u(4))*(max_DFload - min_DFload) + min_DFload;

out(5) = (u(5))*(max_Pa - min_Pa) + min_Pa;

out(6) = (u(6))*(max_Pb - min_Pb) + min_Pb;

out(7) = (u(7))*(max_x - min_x) + min_x;

out(8) = (u(8))*(max_Dx - min_Dx) + min_Dx;

out(9) = (u(9))*(max_Fload - min_Fload) + min_Fload;


y = out;

== matlab function RealLifeTrainModel/DisturbanceEstimationPhase1 ==
  data: f input; g input; current input; dz output; lambda input; F input; z input; dist_model input; gain1 input; gain2 input; Fmenos_z input; intFmenos_z input; dFF input; flag_start input; intintFmenos_z input; gain3 input
function dz = fcn(f,g,current,lambda,F,z,dist_model,gain1,gain2,Fmenos_z,intFmenos_z,dFF,flag_start,intintFmenos_z,gain3)
dz = 0;
if(flag_start == 1)
    if(dist_model == 0)
        dz = (lambda/(g))*(dFF - f - g*current - g*z);
    elseif (dist_model == 1)
        dz = -(lambda*z/(g))*(g) - (lambda/(g))*(lambda*F + f + g*current);
    elseif (dist_model == 2)
        dz = (1/(g))*(f + g*current) + gain1*(Fmenos_z) + gain2*(intFmenos_z) + gain3*intintFmenos_z;
    else
        dz = -(lambda*z) - (lambda)*(lambda*F + f + g*current);
    end
else
    dz = 0;
end

== matlab function RealLifeTrainModel/ContractionMetricFilterSystem3/CalcK/IndidualGrad2/Policy_SS1/FLcontroller1 ==
  data: pid input; y output; f input; g input; dFref input; d input; flag_start input
function y = fcn(pid,f,g,dFref,d,flag_start)

if flag_start == 1
    y = (dFref + pid - f)/g - d;
else 
    y = 1;
end

== matlab function RealLifeTrainModel/ContractionMetricFilterSystem3/CalcK/IndidualGrad2/Policy_SS1/FunctionCalculateHydModel1 ==
  data: ixv input; f output; Pn input; Qn input; Un input; Vpl input; Ps input; Pt input; L_cyl input; Aa input; alfa input; c1 input; c2 input; Be input; flag_start input; data input; g output; force output
function [f,g,force] = fcn(ixv,Pn,Qn,Un,Vpl,Ps,Pt,L_cyl,Aa,alfa,c1,c2,Be,flag_start,data)
force = 0
if flag_start == 1
    Pa = data(5)
    Pb = data(6)
    xp = data(7)
    xpd = data(8)
    force = data(3)

    Kv = Qn/(Un*sqrt(Pn/2));
    
    Va = Vpl + Aa*xp;
    Vb = Vpl + (L_cyl - xp)*alfa*Aa;

    if(ixv >= 0)
        g = Be*Aa*Kv*( sign(Ps-Pa)*sqrt(abs(Ps-Pa))/Va + alfa*sign(Pb-Pt)*sqrt(abs(Pb-Pt))/Vb);
    else
        g = Be*Aa*Kv*( sign(Pa-Pt)*sqrt(abs(Pa-Pt))/Va + alfa*sign(Ps-Pb)*sqrt(abs(Ps-Pb))/Vb);
    end
    
    %g1 = Be*Aa*Kv*( sign(Ps-Pa)*sqrt(abs(Ps-Pa))/Va + alfa*sign(Pb-Pt)*sqrt(abs(Pb-Pt))/Vb);
    %g2 = Be*Aa*Kv*( sign(Pa-Pt)*sqrt(abs(Pa-Pt))/Va + alfa*sign(Ps-Pb)*sqrt(abs(Ps-Pb))/Vb);
    %g = (g1 + g2)/2;

    f = -Be*Aa^2*(((alfa)^2)/Vb + 1/Va)*xpd;
    
    g = c2*g;
    f = c1*f;
    
else
    f = 1;
    g = 1;
end

== matlab function RealLifeTrainModel/ContractionMetricFilterSystem3/CalcK/IndidualGrad2/Policy_SS1/Policy ==
  data: u input; y output
function y = fcn(u)

y = (u)/2 + 0.5;

== matlab function RealLifeTrainModel/ContractionMetricFilterSystem3/CalcK/IndidualGrad2/Policy_SS1/SmoothFnc1 ==
  data: u input; y output; smooth input
function y = fcn(u,smooth)
persistent last_value;

if(isempty(last_value))
    last_value = 0
end

y = smooth*last_value + (1 - smooth)*u
last_value = u

== matlab function RealLifeTrainModel/ContractionMetricFilterSystem3/CalcK/IndidualGrad3/MATLAB Function2 ==
  data: u input; y output; pos input
function y = fcn(u,pos)

a = [0,0,0,0,0,0,0,0,0]

a(pos) = u

y = a;

== matlab function RealLifeTrainModel/ContractionMetricFilterSystem3/CalcK/IndidualGrad3/MATLAB Function5 ==
  data: u1 input; y output; u2 input; const input
function y = fcn(u1,u2,const)

y = (u1 - u2)/(const);

== matlab function RealLifeTrainModel/ContractionMetricFilterSystem3/CalcK/IndidualGrad3/Policy_SS1/Denormalize_Policy ==
  data: u input; y output
function y = fcn(u)

max_Fload =  569.629505294963
min_Fload = -610.339671010468

max_Fhyd = 729.261146885585
min_Fhyd = -777.489547410502

max_DFload = 123011.265014651
min_DFload = -142353.177843906

max_DFhyd = 219994.429294316
min_DFhyd = -270882.694509076

max_Pa = 12037835.3221229
min_Pa = 1849925.22965178

max_Pb = 14831789.6053956
min_Pb = 2808786.27887814

max_x = 0.082368752
min_x = 0.01990812

max_Dx = 0.682789396628826
min_Dx = -0.578996654196926

out = [1,1,1,1,1,1,1,1,1]

out(1) = (u(1))*(max_Fhyd - min_Fhyd) + min_Fhyd;

out(2) = (u(2))*(max_DFhyd - min_DFhyd) + min_DFhyd;

out(3) = (u(3))*(max_Fload - min_Fload) + min_Fload;

out(4) = (u(4))*(max_DFload - min_DFload) + min_DFload;

out(5) = (u(5))*(max_Pa - min_Pa) + min_Pa;

out(6) = (u(6))*(max_Pb - min_Pb) + min_Pb;

out(7) = (u(7))*(max_x - min_x) + min_x;

out(8) = (u(8))*(max_Dx - min_Dx) + min_Dx;

out(9) = (u(9))*(max_Fload - min_Fload) + min_Fload;


y = out;

== matlab function RealLifeTrainModel/ContractionMetricFilterSystem3/CalcK/IndidualGrad3/Policy_SS1/FLcontroller1 ==
  data: pid input; y output; f input; g input; dFref input; d input; flag_start input
function y = fcn(pid,f,g,dFref,d,flag_start)

if flag_start == 1
    y = (dFref + pid - f)/g - d;
else 
    y = 1;
end

== matlab function RealLifeTrainModel/ContractionMetricFilterSystem3/CalcK/IndidualGrad3/Policy_SS1/FunctionCalculateHydModel1 ==
  data: ixv input; f output; Pn input; Qn input; Un input; Vpl input; Ps input; Pt input; L_cyl input; Aa input; alfa input; c1 input; c2 input; Be input; flag_start input; data input; g output; force output
function [f,g,force] = fcn(ixv,Pn,Qn,Un,Vpl,Ps,Pt,L_cyl,Aa,alfa,c1,c2,Be,flag_start,data)
force = 0
if flag_start == 1
    Pa = data(5)
    Pb = data(6)
    xp = data(7)
    xpd = data(8)
    force = data(3)

    Kv = Qn/(Un*sqrt(Pn/2));
    
    Va = Vpl + Aa*xp;
    Vb = Vpl + (L_cyl - xp)*alfa*Aa;

    if(ixv >= 0)
        g = Be*Aa*Kv*( sign(Ps-Pa)*sqrt(abs(Ps-Pa))/Va + alfa*sign(Pb-Pt)*sqrt(abs(Pb-Pt))/Vb);
    else
        g = Be*Aa*Kv*( sign(Pa-Pt)*sqrt(abs(Pa-Pt))/Va + alfa*sign(Ps-Pb)*sqrt(abs(Ps-Pb))/Vb);
    end
    
    %g1 = Be*Aa*Kv*( sign(Ps-Pa)*sqrt(abs(Ps-Pa))/Va + alfa*sign(Pb-Pt)*sqrt(abs(Pb-Pt))/Vb);
    %g2 = Be*Aa*Kv*( sign(Pa-Pt)*sqrt(abs(Pa-Pt))/Va + alfa*sign(Ps-Pb)*sqrt(abs(Ps-Pb))/Vb);
    %g = (g1 + g2)/2;

    f = -Be*Aa^2*(((alfa)^2)/Vb + 1/Va)*xpd;
    
    g = c2*g;
    f = c1*f;
    
else
    f = 1;
    g = 1;
end

== matlab function RealLifeTrainModel/ContractionMetricFilterSystem3/CalcK/IndidualGrad3/Policy_SS1/Policy ==
  data: u input; y output
function y = fcn(u)

y = (u)/2 + 0.5;

== matlab function RealLifeTrainModel/ContractionMetricFilterSystem3/CalcK/IndidualGrad3/Policy_SS1/SmoothFnc1 ==
  data: u input; y output; smooth input
function y = fcn(u,smooth)
persistent last_value;

if(isempty(last_value))
    last_value = 0
end

y = smooth*last_value + (1 - smooth)*u
last_value = u

== matlab function RealLifeTrainModel/ContractionMetricFilterSystem3/CalcK/IndidualGrad4/MATLAB Function2 ==
  data: u input; y output; pos input
function y = fcn(u,pos)

a = [0,0,0,0,0,0,0,0,0]

a(pos) = u

y = a;

== matlab function RealLifeTrainModel/ContractionMetricFilterSystem3/CalcK/IndidualGrad4/MATLAB Function5 ==
  data: u1 input; y output; u2 input; const input
function y = fcn(u1,u2,const)

y = (u1 - u2)/(const);

== matlab function RealLifeTrainModel/ContractionMetricFilterSystem3/CalcK/IndidualGrad4/Policy_SS1/Denormalize_Policy ==
  data: u input; y output
function y = fcn(u)

max_Fload =  569.629505294963
min_Fload = -610.339671010468

max_Fhyd = 729.261146885585
min_Fhyd = -777.489547410502

max_DFload = 123011.265014651
min_DFload = -142353.177843906

max_DFhyd = 219994.429294316
min_DFhyd = -270882.694509076

max_Pa = 12037835.3221229
min_Pa = 1849925.22965178

max_Pb = 14831789.6053956
min_Pb = 2808786.27887814

max_x = 0.082368752
min_x = 0.01990812

max_Dx = 0.682789396628826
min_Dx = -0.578996654196926

out = [1,1,1,1,1,1,1,1,1]

out(1) = (u(1))*(max_Fhyd - min_Fhyd) + min_Fhyd;

out(2) = (u(2))*(max_DFhyd - min_DFhyd) + min_DFhyd;

out(3) = (u(3))*(max_Fload - min_Fload) + min_Fload;

out(4) = (u(4))*(max_DFload - min_DFload) + min_DFload;

out(5) = (u(5))*(max_Pa - min_Pa) + min_Pa;

out(6) = (u(6))*(max_Pb - min_Pb) + min_Pb;

out(7) = (u(7))*(max_x - min_x) + min_x;

out(8) = (u(8))*(max_Dx - min_Dx) + min_Dx;

out(9) = (u(9))*(max_Fload - min_Fload) + min_Fload;


y = out;

== matlab function RealLifeTrainModel/ContractionMetricFilterSystem3/CalcK/IndidualGrad4/Policy_SS1/FLcontroller1 ==
  data: pid input; y output; f input; g input; dFref input; d input; flag_start input
function y = fcn(pid,f,g,dFref,d,flag_start)

if flag_start == 1
    y = (dFref + pid - f)/g - d;
else 
    y = 1;
end

== matlab function RealLifeTrainModel/ContractionMetricFilterSystem3/CalcK/IndidualGrad4/Policy_SS1/FunctionCalculateHydModel1 ==
  data: ixv input; f output; Pn input; Qn input; Un input; Vpl input; Ps input; Pt input; L_cyl input; Aa input; alfa input; c1 input; c2 input; Be input; flag_start input; data input; g output; force output
function [f,g,force] = fcn(ixv,Pn,Qn,Un,Vpl,Ps,Pt,L_cyl,Aa,alfa,c1,c2,Be,flag_start,data)
force = 0
if flag_start == 1
    Pa = data(5)
    Pb = data(6)
    xp = data(7)
    xpd = data(8)
    force = data(3)

    Kv = Qn/(Un*sqrt(Pn/2));
    
    Va = Vpl + Aa*xp;
    Vb = Vpl + (L_cyl - xp)*alfa*Aa;

    if(ixv >= 0)
        g = Be*Aa*Kv*( sign(Ps-Pa)*sqrt(abs(Ps-Pa))/Va + alfa*sign(Pb-Pt)*sqrt(abs(Pb-Pt))/Vb);
    else
        g = Be*Aa*Kv*( sign(Pa-Pt)*sqrt(abs(Pa-Pt))/Va + alfa*sign(Ps-Pb)*sqrt(abs(Ps-Pb))/Vb);
    end
    
    %g1 = Be*Aa*Kv*( sign(Ps-Pa)*sqrt(abs(Ps-Pa))/Va + alfa*sign(Pb-Pt)*sqrt(abs(Pb-Pt))/Vb);
    %g2 = Be*Aa*Kv*( sign(Pa-Pt)*sqrt(abs(Pa-Pt))/Va + alfa*sign(Ps-Pb)*sqrt(abs(Ps-Pb))/Vb);
    %g = (g1 + g2)/2;

    f = -Be*Aa^2*(((alfa)^2)/Vb + 1/Va)*xpd;
    
    g = c2*g;
    f = c1*f;
    
else
    f = 1;
    g = 1;
end

== matlab function RealLifeTrainModel/ContractionMetricFilterSystem3/CalcK/IndidualGrad4/Policy_SS1/Policy ==
  data: u input; y output
function y = fcn(u)

y = (u)/2 + 0.5;

== matlab function RealLifeTrainModel/ContractionMetricFilterSystem3/CalcK/IndidualGrad4/Policy_SS1/SmoothFnc1 ==
  data: u input; y output; smooth input
function y = fcn(u,smooth)
persistent last_value;

if(isempty(last_value))
    last_value = 0
end

y = smooth*last_value + (1 - smooth)*u
last_value = u

== matlab function RealLifeTrainModel/ContractionMetricFilterSystem3/CalcK/IndidualGrad5/MATLAB Function2 ==
  data: u input; y output; pos input
function y = fcn(u,pos)

a = [0,0,0,0,0,0,0,0,0]
a(pos) = u

y = a;

== matlab function RealLifeTrainModel/FLcontroller ==
  data: pid input; y output; f input; g input; dFref input; d input; flag_start input
function y = fcn(pid,f,g,dFref,d,flag_start)

if flag_start == 1
    y = (dFref + pid - f)/g - d;
else 
    y = 1;
end

== matlab function RealLifeTrainModel/ContractionMetricFilterSystem3/CalcK/IndidualGrad5/MATLAB Function5 ==
  data: u1 input; y output; u2 input; const input
function y = fcn(u1,u2,const)

y = (u1 - u2)/(const);

== matlab function RealLifeTrainModel/ContractionMetricFilterSystem3/CalcK/IndidualGrad5/Policy_SS1/Denormalize_Policy ==
  data: u input; y output
function y = fcn(u)

max_Fload =  569.629505294963
min_Fload = -610.339671010468

max_Fhyd = 729.261146885585
min_Fhyd = -777.489547410502

max_DFload = 123011.265014651
min_DFload = -142353.177843906

max_DFhyd = 219994.429294316
min_DFhyd = -270882.694509076

max_Pa = 12037835.3221229
min_Pa = 1849925.22965178

max_Pb = 14831789.6053956
min_Pb = 2808786.27887814

max_x = 0.082368752
min_x = 0.01990812

max_Dx = 0.682789396628826
min_Dx = -0.578996654196926

out = [1,1,1,1,1,1,1,1,1]

out(1) = (u(1))*(max_Fhyd - min_Fhyd) + min_Fhyd;

out(2) = (u(2))*(max_DFhyd - min_DFhyd) + min_DFhyd;

out(3) = (u(3))*(max_Fload - min_Fload) + min_Fload;

out(4) = (u(4))*(max_DFload - min_DFload) + min_DFload;

out(5) = (u(5))*(max_Pa - min_Pa) + min_Pa;

out(6) = (u(6))*(max_Pb - min_Pb) + min_Pb;

out(7) = (u(7))*(max_x - min_x) + min_x;

out(8) = (u(8))*(max_Dx - min_Dx) + min_Dx;

out(9) = (u(9))*(max_Fload - min_Fload) + min_Fload;


y = out;

== matlab function RealLifeTrainModel/ContractionMetricFilterSystem3/CalcK/IndidualGrad5/Policy_SS1/FLcontroller1 ==
  data: pid input; y output; f input; g input; dFref input; d input; flag_start input
function y = fcn(pid,f,g,dFref,d,flag_start)

if flag_start == 1
    y = (dFref + pid - f)/g - d;
else 
    y = 1;
end

== matlab function RealLifeTrainModel/ContractionMetricFilterSystem3/CalcK/IndidualGrad5/Policy_SS1/FunctionCalculateHydModel1 ==
  data: ixv input; f output; Pn input; Qn input; Un input; Vpl input; Ps input; Pt input; L_cyl input; Aa input; alfa input; c1 input; c2 input; Be input; flag_start input; data input; g output; force output
function [f,g,force] = fcn(ixv,Pn,Qn,Un,Vpl,Ps,Pt,L_cyl,Aa,alfa,c1,c2,Be,flag_start,data)
force = 0
if flag_start == 1
    Pa = data(5)
    Pb = data(6)
    xp = data(7)
    xpd = data(8)
    force = data(3)

    Kv = Qn/(Un*sqrt(Pn/2));
    
    Va = Vpl + Aa*xp;
    Vb = Vpl + (L_cyl - xp)*alfa*Aa;

    if(ixv >= 0)
        g = Be*Aa*Kv*( sign(Ps-Pa)*sqrt(abs(Ps-Pa))/Va + alfa*sign(Pb-Pt)*sqrt(abs(Pb-Pt))/Vb);
    else
        g = Be*Aa*Kv*( sign(Pa-Pt)*sqrt(abs(Pa-Pt))/Va + alfa*sign(Ps-Pb)*sqrt(abs(Ps-Pb))/Vb);
    end
    
    %g1 = Be*Aa*Kv*( sign(Ps-Pa)*sqrt(abs(Ps-Pa))/Va + alfa*sign(Pb-Pt)*sqrt(abs(Pb-Pt))/Vb);
    %g2 = Be*Aa*Kv*( sign(Pa-Pt)*sqrt(abs(Pa-Pt))/Va + alfa*sign(Ps-Pb)*sqrt(abs(Ps-Pb))/Vb);
    %g = (g1 + g2)/2;

    f = -Be*Aa^2*(((alfa)^2)/Vb + 1/Va)*xpd;
    
    g = c2*g;
    f = c1*f;
    
else
    f = 1;
    g = 1;
end

== matlab function RealLifeTrainModel/ContractionMetricFilterSystem3/CalcK/IndidualGrad5/Policy_SS1/Policy ==
  data: u input; y output
function y = fcn(u)

y = (u)/2 + 0.5;

== matlab function RealLifeTrainModel/ContractionMetricFilterSystem3/CalcK/IndidualGrad5/Policy_SS1/SmoothFnc1 ==
  data: u input; y output; smooth input
function y = fcn(u,smooth)
persistent last_value;

if(isempty(last_value))
    last_value = 0
end

y = smooth*last_value + (1 - smooth)*u
last_value = u

== matlab function RealLifeTrainModel/ContractionMetricFilterSystem3/CalcK/IndidualGrad6/MATLAB Function2 ==
  data: u input; y output; pos input
function y = fcn(u,pos)

a = [0,0,0,0,0,0,0,0,0]

a(pos) = u

y = a;

== matlab function RealLifeTrainModel/ContractionMetricFilterSystem3/CalcK/IndidualGrad6/MATLAB Function5 ==
  data: u1 input; y output; u2 input; const input
function y = fcn(u1,u2,const)

y = (u1 - u2)/(const);
